simulink model "Q8_Model"  (R2025b)
settings: Solver=VariableStepAuto  StartTime=0.0  StopTime=10.0  RelTol=1e-3
values from neighbouring files (symbols this model uses):
  A_Q8 = A - B*K - L*C    [main.m]
  D = [0 0]'    [main.m]
  K = lqr(A, B, Qr, Rr)    [IP_MACRO.m]
  L = lqe(A, G, C, Qe, Re)    [IP_MACRO.m]    (also in main.m)
  x0 = [0.1 0 0 0 0]'    [main.m]
undefined symbols (not defined in the file or in its folder): A, B, C
settings Model: Creator=lucas  LastModifiedBy=texman

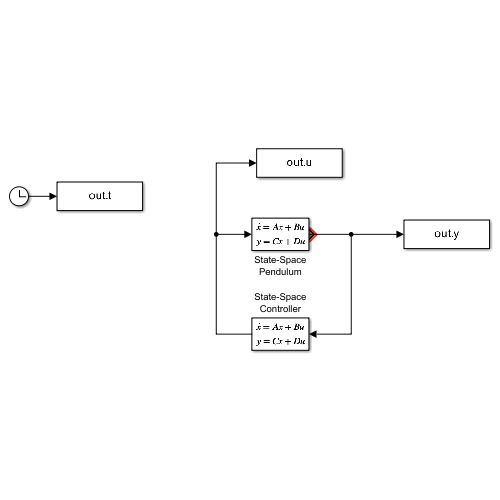
[thumbnail: Simulink's stored preview of the top-level diagram]
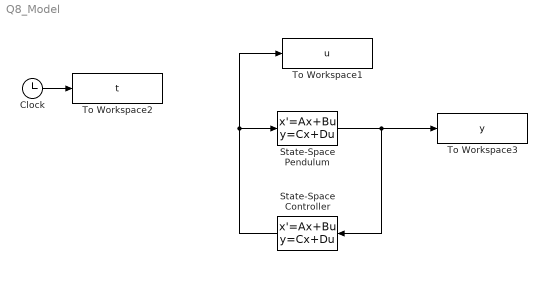
== system Q8_Model ==
  Clock : Clock
  State-Space Controller : StateSpace  A=A_Q8  B=L  C=-K  D=[0 0]  InitialCondition=0  ParameterTunability=Unconstrained  ContinuousStateAttributes={'y1','y2','y3','y4','y5'}
  State-Space Pendulum : StateSpace  A=A  B=B  C=C  D=D  InitialCondition=x0  ContinuousStateAttributes={'x1','x2','x3','x4','x5'}
  To Workspace1 : ToWorkspace  VariableName=u  SaveFormat=Timeseries  SampleTime=-1
  To Workspace2 : ToWorkspace  VariableName=t  SaveFormat=Timeseries  SampleTime=-1
  To Workspace3 : ToWorkspace  VariableName=y  SaveFormat=Timeseries  SampleTime=-1
  wires:
  State-Space Pendulum/1 -> To Workspace3/1, State-Space Controller/1
  State-Space Controller/1 -> To Workspace1/1, State-Space Pendulum/1
  Clock/1 -> To Workspace2/1
